simulink model "WATER_TASK1_MAIN"  (R2024b)
settings: Solver=VariableStepAuto  StartTime=0.0  StopTime=300  RelTol=1e-3
settings Model: Creator=Dharmesh  LastModifiedBy=Dharmesh

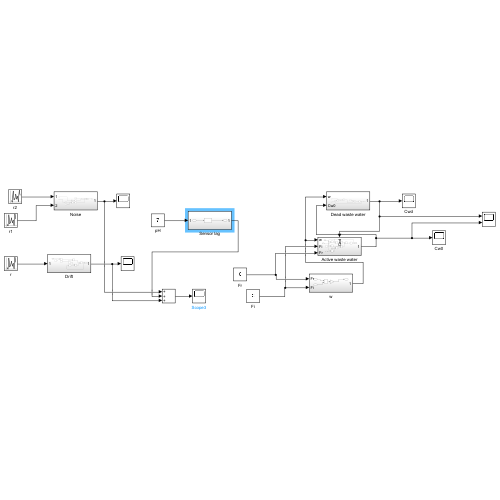
[thumbnail: Simulink's stored preview of the top-level diagram]
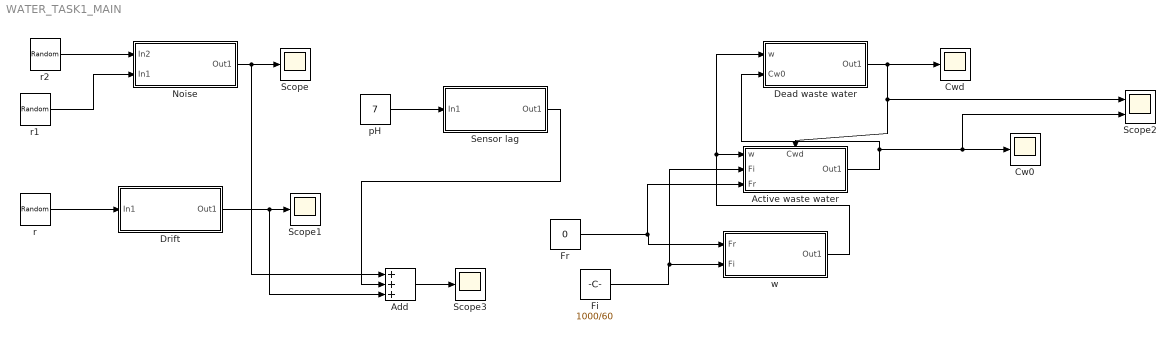
== system WATER_TASK1_MAIN ==
  Active waste water : Subsystem
      settings: PortSchema="{\"entries\":[{\"content\":{\"sides\":[{\"content\":{\"connectorIds\":[\"In1\",\"In2\",\"In3\"]},\"type\":\"ConnectorPlacement.EquallySpacedRectSide\",\"uuid\":\"fdd08be6-e542-434b-bcfd-e03d8eb8934a\"},{\"content\":{\"connectorIds\":[\"Out1\"],\"side\":\"RIGHT\"},\"type\":\"ConnectorPlacement.EquallySpacedRectSide\",\"uuid\":\"3363dfa2-2fb6-4b70-9eec-cac1e7b4f1e0\"},{\"content\":{\"connectorIds\":[\"In4\"],\"side\":\"TOP\"},\"type\":\"ConnectorPlacement.EquallySpacedRectSide\",\"uuid\":\"b10648a6-2485-4102-8fdc-da396d8924bf\"}]},\"type\":\"ConnectorPlacement.EquallySpacedConnector\",\"uuid\":\"036e3afb-3366-4cdb-9c6c-a79e45bd74a4\"}],\"packageUris\":[\"http://schema.mathworks.com/mf0/Connector/R2020b\"],\"version\":\"1.0\"}"
  Add : Sum  Inputs=+++
  Cw0 : Scope
  Cwd : Scope
  Dead waste water : Subsystem
  Drift : Subsystem
  Fi : Constant  Value=1000/60
  Fr : Constant  Value=0
  Noise : Subsystem
  Scope : Scope
  Scope1 : Scope
  Scope2 : Scope  NumInputPorts=2
  Scope3 : Scope
  Sensor lag : Subsystem
  pH : Constant  Value=7
  r : UniformRandomNumber  Minimum=0  SampleTime=0.1
  r1 : UniformRandomNumber  Minimum=0.000001  SampleTime=0.1
  r2 : UniformRandomNumber  Minimum=0  SampleTime=0.1
  w : Subsystem
  wires:
  r2/1 -> Noise/1(In2)
  r1/1 -> Noise/2(In1)
  Noise/1(Out1) -> Add/1, Scope/1
  r/1 -> Drift/1(In1)
  Drift/1(Out1) -> Add/3, Scope1/1
  Dead waste water/1(Out1) -> Active waste water/4(Cwd), Scope2/1, Cwd/1
  Active waste water/1(Out1) -> Scope2/2, Cw0/1, Dead waste water/2(Cw0)
  Fr/1 -> Active waste water/3(Fr), w/1(Fr)
  Fi/1 -> Active waste water/2(Fi), w/2(Fi)
  w/1(Out1) -> Dead waste water/1(w), Active waste water/1(w)
  pH/1 -> Sensor lag/1(In1)
  Sensor lag/1(Out1) -> Add/2
  Add/1 -> Scope3/1

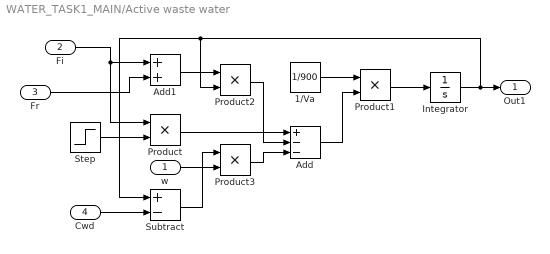
== system WATER_TASK1_MAIN/Active waste water ==
  w : Inport
  Fi : Inport  Port=2
  Fr : Inport  Port=3
  Cwd : Inport  Port=4
  1/Va : Constant  Value=1/900
  Add : Sum  Inputs=+--
  Add1 : Sum
  Integrator : Integrator  InitialCondition=0.001
  Product{,1..3} (4 alike) : Product
  Step : Step  Time=20  Before=0.001  After=0  SampleTime=0
  Subtract : Sum  Inputs=+-
  Out1 : Outport
  wires:
  Fi/1 -> Add1/1, Product/1
  Product/1 -> Add/1
  Fr/1 -> Add1/2
  w/1 -> Product3/2
  Step/1 -> Product/2
  Cwd/1 -> Subtract/2
  Add/1 -> Product1/2
  Add1/1 -> Product2/1
  Subtract/1 -> Product3/1
  Product2/1 -> Add/2
  1/Va/1 -> Product1/1
  Product3/1 -> Add/3
  Product1/1 -> Integrator/1
  Integrator/1 -> Subtract/1, Product2/2, Out1/1

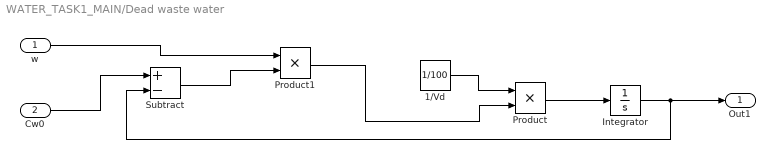
== system WATER_TASK1_MAIN/Dead waste water ==
  w : Inport
  Cw0 : Inport  Port=2
  1/Vd : Constant  Value=1/100
  Integrator : Integrator  InitialCondition=0.001
  Product : Product
  Product1 : Product
  Subtract : Sum  Inputs=+-
  Out1 : Outport
  wires:
  Integrator/1 -> Subtract/2, Out1/1
  Product/1 -> Integrator/1
  1/Vd/1 -> Product/1
  Cw0/1 -> Subtract/1
  Subtract/1 -> Product1/2
  w/1 -> Product1/1
  Product1/1 -> Product/2

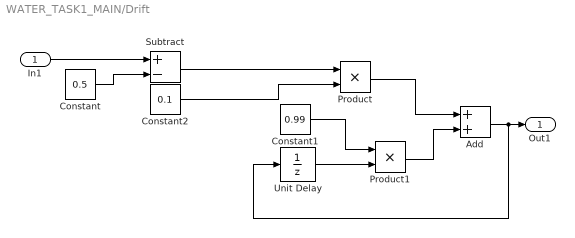
== system WATER_TASK1_MAIN/Drift ==
  In1 : Inport
  Add : Sum
  Constant : Constant  Value=0.5
  Constant1 : Constant  Value=0.99
  Constant2 : Constant  Value=0.1
  Product : Product
  Product1 : Product
  Subtract : Sum  Inputs=+-
  Unit Delay : UnitDelay  SampleTime=-1  HasFrameUpgradeWarning=on
  Out1 : Outport
  wires:
  Add/1 -> Unit Delay/1, Out1/1
  In1/1 -> Subtract/1
  Constant/1 -> Subtract/2
  Subtract/1 -> Product/1
  Constant2/1 -> Product/2
  Unit Delay/1 -> Product1/2
  Constant1/1 -> Product1/1
  Product/1 -> Add/1
  Product1/1 -> Add/2

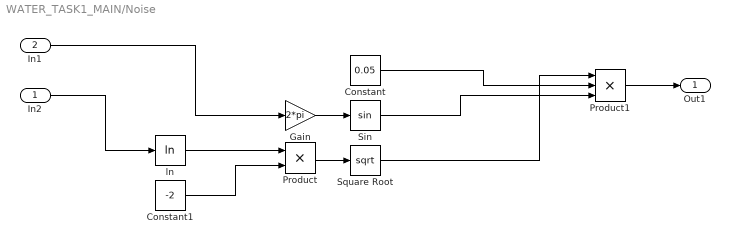
== system WATER_TASK1_MAIN/Noise ==
  In2 : Inport
  In1 : Inport  Port=2
  Constant : Constant  Value=0.05
  Constant1 : Constant  Value=-2
  Gain : Gain  Gain=2*pi
  Product : Product
  Product1 : Product  Inputs=3
  Sin : Trigonometry
  Square Root : Sqrt
  ln : Math  Operator=log
  Out1 : Outport
  wires:
  In1/1 -> Gain/1
  In2/1 -> ln/1
  Square Root/1 -> Product1/1
  ln/1 -> Product/1
  Constant/1 -> Product1/2
  Product/1 -> Square Root/1
  Constant1/1 -> Product/2
  Sin/1 -> Product1/3
  Gain/1 -> Sin/1
  Product1/1 -> Out1/1

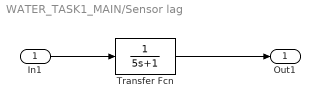
== system WATER_TASK1_MAIN/Sensor lag ==
  In1 : Inport
  Transfer Fcn : TransferFcn  Denominator=[5 1]
  Out1 : Outport
  wires:
  In1/1 -> Transfer Fcn/1
  Transfer Fcn/1 -> Out1/1

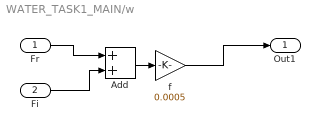
== system WATER_TASK1_MAIN/w ==
  Fr : Inport
  Fi : Inport  Port=2
  Add : Sum
  f : Gain  Gain=0.0005
  Out1 : Outport
  wires:
  Fr/1 -> Add/1
  Fi/1 -> Add/2
  Add/1 -> f/1
  f/1 -> Out1/1
